simulink model "DC_Motor_Characteristcs"  (R2017a)
settings: Solver=FixedStepAuto  StartTime=0.0  StopTime=300  MaxStep=1e-4  RelTol=1e-3
StopFcn:
  | figure();
  | plot(Ia.Data,W.Data);
  | xlabel('Armature Current');
  | ylabel('Speed');
  | title('Shut Motor Characteristics')
  | 
  | figure();
  | plot(Ia.Data,T.Data);
  | xlabel('Armature Current');
  | ylabel('Torque');
  | title('Shut Motor Characteristics');
  | 
  | figure();
  | plot(Ia1.Data,W1.Data);
  | xlabel('Armature Current');
  | ylabel('Speed');
  | title('Series Motor Characteristics')
  | 
  | figure();
  | plot(Ia1.Data,T1.Data);
  | xlabel('Armature Current');
  | ylabel('Torque');
  | title('Series Motor Characteristics');
libraries: powerlib x3, simulink x1
settings Model: Creator=satendra  LastModifiedBy=satendra

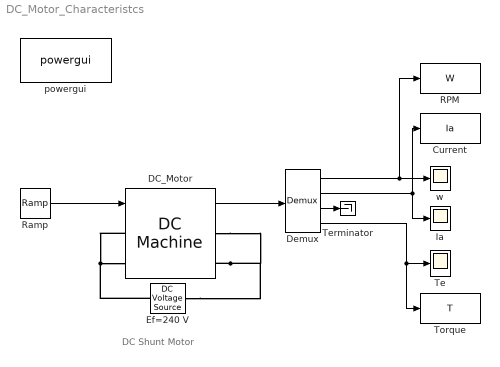
== system DC_Motor_Characteristcs ==
  note: DC Shunt Motor
  Current : ToWorkspace  VariableName=Ia  SaveFormat=Timeseries  SampleTime=-1
  "DC_Motor " : powerlib/Machines/DC Machine  PresetModel=01: 5HP 240V 1750RPM Field:300V  MechanicalLoad=Torque TL  FieldType=Wound  ShowDetailedParameters=on  MeasurementBus=off  RLa=[2.581 0.028]  RLf=[281.3 156]  Laf=0.9483  MachineConstant=Torque constant (N.m/A)  Ke=1.8  Kt=1.8  J=0.02215  Bm=0.002953  Tf=0.5161  w0=1  Ifinit=1  TsPowergui=0  TsBlock=-1
      settings: AttributesFormatString=\n
  Demux : Demux
  Ef=240 V : powerlib/Electrical Sources/DC Voltage Source  Description=source block  Amplitude=240  Measurements=None
      settings: AttributesFormatString=\n
  Ia : Scope
  RPM : ToWorkspace  VariableName=W  SaveFormat=Timeseries  SampleTime=-1
  Ramp : simulink/Sources/Ramp  slope=1  start=0  X0=0
  Te : Scope
  Terminator : Terminator
  Torque : ToWorkspace  VariableName=T  SaveFormat=Timeseries  SampleTime=-1
  powergui : powerlib/powergui  Priority=2  SimulationMode=Discrete  SampleTime=50e-6  frequency=60  Iterations=50  frequencyindice=0  Pbase=100e6  ErrMax=1e-4  UnitsV=kV  UnitsW=MW  buscounter=0  FunctionMessages=off  echomessages=off  EnableUseOfTLC=off  CurrentSourceSwitches=off  DisableSnubberDevices=off  DisableRonSwitches=off  DisableVfSwitches=off  DisplayEquations=off  SolverType=Tustin/Backward Euler (TBE)  Interpol=off  ExternalGateDelay=off  methode=off  Ts=100  x0status=blocks  SPID=off  SwTol=0  HookPort=off  RestoreLinks=warning  ResistiveCurrentMeasurement=off  Frange=logspace(0,3,50)  Ylog=off  Xlog=off  ShowGrid=off  save=off  variable=ZData  structure=0  ZoomFFT=on  StartTime=0.0  cycles=1  DisplayStyle=off  fundamental=60  FreqAxis=off  MaxFrequency=1000  frequencyindicesteady=1  RmsSteady=1  display=off
  w : Scope
  wires:
  Demux/2 -> Ia/1, Current/1
  Demux/1 -> RPM/1, w/1
  "DC_Motor "/1 -> Demux/1
  Demux/3 -> Terminator/1
  Ramp/1 -> "DC_Motor "/1
  Demux/4 -> Torque/1, Te/1
  connections:
  "DC_Motor "/RConn2 -- Ef=240 V/LConn1 -- "DC_Motor "/RConn1
  Ef=240 V/RConn1 -- "DC_Motor "/LConn1 -- "DC_Motor "/LConn2
